simulink model "DLCReferenceApplication"  (R2018a)
settings: Solver=ode23tb  StartTime=0.0  StopTime=20  FixedStep=.001  RelTol=5e-3  EnableMultiTasking=on
StartFcn:
  | %tic
StopFcn:
  | %toc
model workspace (MAT data in the model file):
  A_mu = 10
  B_reff = 8.386
  Cz = 7766.25
  DCT_Param : struct (value not decoded)
  D_reff = 0.25826
  Downshift_Speeds = [9.5625 12.9375 16.3125 19.6875 23.0625 26.4375 29.8125 33.1875 36.5625 39.9375 43.3125 46.6875 ... (28 elements, 4x7)]
  Pedal_Positions = [0.1 0.4 0.5 0.9]
  SUS : struct (value not decoded)
  Upshift_Speeds = [12.9375 16.3125 19.6875 33 26.4375 29.8125 33.1875 52.5 39.9375 43.3125 46.6875 77.25 ... (28 elements, 4x7)]
  VEH : struct (value not decoded)
  V_o = 16.7
  V_xlow = 1
  WH : struct (value not decoded)
  a = 1.4
  alpha_max = 1.5
  alpha_min = -1.5
  b = 1.8
  c_zo = 209651
  epsilon = 0.1
  h = 0.134
  path : struct (value not decoded)
  pio = 220000
  q_Fcx = 0
  q_Fz2 = 15.4
  q_Fzy = 0
  q_reo = 0.9974
  q_sx1 = -0.007764
  q_sx10 = 0.2824
  q_sx11 = 5.349
  q_sx12 = 0
  q_sx13 = 0
  q_sx14 = 0
  q_sx2 = 1.1915
  q_sx3 = 0.013948
  q_sx4 = 4.912
  q_sx5 = 1.02
  q_sx6 = 22.83
  q_sx7 = 0.7104
  q_sx8 = -0.023393
  q_sx9 = 0.6581
  q_sy1 = 0.00702
  q_sy2 = 0
  q_sy3 = 0.001515
  q_sy4 = 8.514e-05
  q_sy5 = 0
  q_sy6 = 0
  q_sy7 = 0.9008
  q_sy8 = -0.4089
  q_v1 = 0.0007742
  q_v2 = 0.04667
  r_Bx1 = 12.531
  r_Bx2 = 9.532
  r_Bx3 = 0
  r_By1 = 10.615
  r_By2 = 7.705
  r_By3 = 3.433e-06
  r_By4 = 0
  r_Cx1 = 1.019
  r_Cy1 = 1.0585
  r_Ex1 = -0.4487
  r_Ex2 = -0.4726
  r_Ey1 = 0.3132
  r_Ey2 = 7.63e-06
  r_Hx1 = 0.0002374
  r_Hy1 = 0.011646
  r_Hy2 = 7.63e-06
  r_Vy1 = 0.05654
  r_Vy2 = 7.63e-06
  r_Vy3 = 0
  r_Vy4 = 99.9
  r_Vy5 = 2
  r_Vy6 = 15.814
  r_o = 0.3135
  vehWidth = 2
  w = 1
symbols that are objects in the model workspace (value not decoded): VEH
libraries: neural x286, simulink x5, sim3dlib x2, autolibutils x1, vehdynlibscenariocommon x1, vehdynlibdriver x1, vehdynlibviscommon x1
(part 8 of 13)

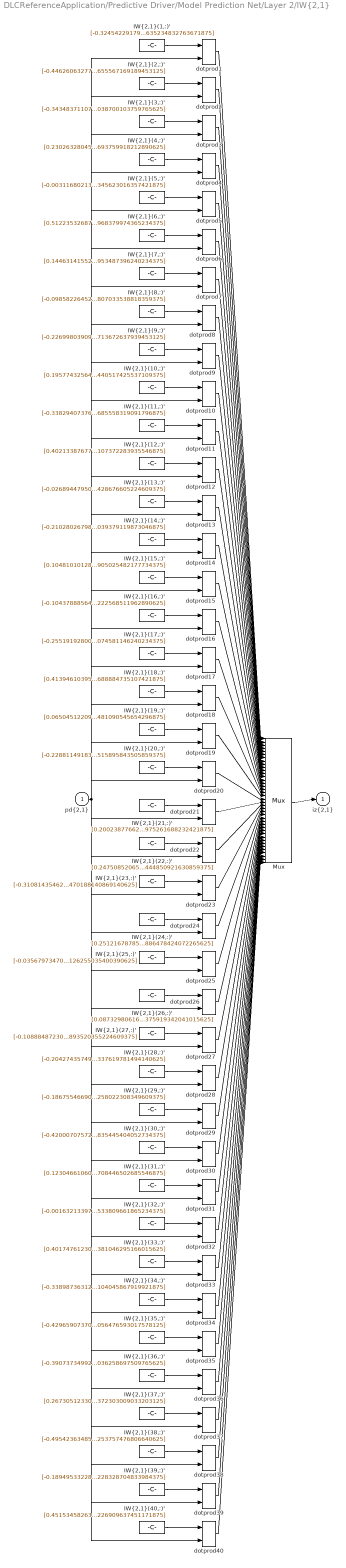
== system DLCReferenceApplication/Predictive Driver/Model Prediction Net/Layer 2/IW{2,1} ==
  "pd{2,1}" : Inport  PortDimensions=9
      mask Display: e = 0.06;c1 = [120 230 180]/255;c2 = ([120 230 180]+0)/(256+128);c3 = ([120 230 180]+128)/(256+128);patch([0 1 1 0],[0 0 1 1],c1);patch([0 1 1 1-e 1-e 0+e],[0 0 1 1-e 0+e 0+e],c2);patch([0 0 1 1-e 0+e 0+e],[0 1 1 1-e 1-e 0+e],c3);plot([0 1 1 0 0],[0 0 1 1 0]);
  "IW{2,1}(1,:)'" : Constant  Value=[-0.324542291796775683732079187393537722527980804443359375;0.0687875470540312006217931184437475167214870452880859375;-0.28041153589947598323561805955250747501850128173828125;0.1679354382406141044103975445977994240820407867431640625;-0.00584034343573799387405731664557606563903391361236572265625;-0.08695050204507125124475663824341609142720699310302734375;-0.37068121178757651446034060427336953580379486083984375;0.63669738948850274073976152067189104855060577392578125;-0.38189062518176353222543184529058635234832763671875]
      mask Display: e = 0.06;c1 = [120 150 230]/255;c2 = ([120 150 230]+0)/383;c3 = ([120 150 230]+128)/383;patch([0 1 1 0],[0 0 1 1],c1);patch([0 1 1 1-e 1-e 0+e],[0 0 1 1-e 0+e 0+e],c2);patch([0 0 1 1-e 0+e 0+e],[0 1 1 1-e 1-e 0+e],c3);plot([0 1 1 0 0],[0 0 1 1 0]);disp('Weights');
  "IW{2,1}(10,:)'" : Constant  Value=[0.1957743256441802082168379683935199864208698272705078125;-0.00790690423303845764391173389640243840403854846954345703125;0.2807004355283073682159056261298246681690216064453125;-0.1709484406753312979443393260226002894341945648193359375;0.1292261121435868409523806121796951629221439361572265625;0.090576606811163140609011179549270309507846832275390625;-0.30742917612599141019558146581402979791164398193359375;0.5389468080432144869718058544094674289226531982421875;-0.355730641305932626661245876675820909440517425537109375]
      mask Display: e = 0.06;c1 = [120 150 230]/255;c2 = ([120 150 230]+0)/383;c3 = ([120 150 230]+128)/383;patch([0 1 1 0],[0 0 1 1],c1);patch([0 1 1 1-e 1-e 0+e],[0 0 1 1-e 0+e 0+e],c2);patch([0 0 1 1-e 0+e 0+e],[0 1 1 1-e 1-e 0+e],c3);plot([0 1 1 0 0],[0 0 1 1 0]);disp('Weights');
  "IW{2,1}(11,:)'" : Constant  Value=[-0.3382940737674229314535523371887393295764923095703125;0.136301301719288614489045130540034733712673187255859375;0.077184732021632618259587843567715026438236236572265625;-0.2946849138566107750847322677145712077617645263671875;0.55020512470717031217048997859819792211055755615234375;0.336723165091655063374531664521782658994197845458984375;-0.496038250235261990450652547224308364093303680419921875;-0.2276057442694929822124549900763668119907379150390625;0.221570869972811113068900112921255640685558319091796875]
      mask Display: e = 0.06;c1 = [120 150 230]/255;c2 = ([120 150 230]+0)/383;c3 = ([120 150 230]+128)/383;patch([0 1 1 0],[0 0 1 1],c1);patch([0 1 1 1-e 1-e 0+e],[0 0 1 1-e 0+e 0+e],c2);patch([0 0 1 1-e 0+e 0+e],[0 1 1 1-e 1-e 0+e],c3);plot([0 1 1 0 0],[0 0 1 1 0]);disp('Weights');
  "IW{2,1}(12,:)'" : Constant  Value=[0.40213387677751477600196494677220471203327178955078125;0.136644910573546829457569629084900952875614166259765625;-0.2578531101404093472950762588880024850368499755859375;0.310418938284677980998793600520002655684947967529296875;-0.4257927265207228639809500236879102885723114013671875;-0.498352245956162509532560989100602455437183380126953125;0.1750266792239182633839078562232316471636295318603515625;-0.00128703269928016048907759572017539539956487715244293212890625;0.49355683974621011866901199027779512107372283935546875]
      mask Display: e = 0.06;c1 = [120 150 230]/255;c2 = ([120 150 230]+0)/383;c3 = ([120 150 230]+128)/383;patch([0 1 1 0],[0 0 1 1],c1);patch([0 1 1 1-e 1-e 0+e],[0 0 1 1-e 0+e 0+e],c2);patch([0 0 1 1-e 0+e 0+e],[0 1 1 1-e 1-e 0+e],c3);plot([0 1 1 0 0],[0 0 1 1 0]);disp('Weights');
  "IW{2,1}(13,:)'" : Constant  Value=[-0.0268944795008402744163067410454459604807198047637939453125;0.160778563268169139011121160365291871130466461181640625;-0.63333375741451813922822111635468900203704833984375;-0.361822351242176265539995938524953089654445648193359375;0.080833836745488218955557613298879005014896392822265625;0.272846015059181545847621919165248982608318328857421875;0.0640400439979145474911348401292343623936176300048828125;-0.4070909764860017876486608656705357134342193603515625;0.2056920660289839053458393891560263000428676605224609375]
      mask Display: e = 0.06;c1 = [120 150 230]/255;c2 = ([120 150 230]+0)/383;c3 = ([120 150 230]+128)/383;patch([0 1 1 0],[0 0 1 1],c1);patch([0 1 1 1-e 1-e 0+e],[0 0 1 1-e 0+e 0+e],c2);patch([0 0 1 1-e 0+e 0+e],[0 1 1 1-e 1-e 0+e],c3);plot([0 1 1 0 0],[0 0 1 1 0]);disp('Weights');
  "IW{2,1}(14,:)'" : Constant  Value=[-0.2102802679827652510002877761507988907396793365478515625;0.3021164324474343576554247192689217627048492431640625;-0.60946876714005371322713244808255694806575775146484375;-0.05831772096079734790663451349246315658092498779296875;0.044852540651126072968057911793948733247816562652587890625;0.51936381618280014205168981789029203355312347412109375;0.39191774273829504959820724252494983375072479248046875;-0.07643630317209677837997361393718165345489978790283203125;0.10716909492530739267390771374266478233039379119873046875]
      mask Display: e = 0.06;c1 = [120 150 230]/255;c2 = ([120 150 230]+0)/383;c3 = ([120 150 230]+128)/383;patch([0 1 1 0],[0 0 1 1],c1);patch([0 1 1 1-e 1-e 0+e],[0 0 1 1-e 0+e 0+e],c2);patch([0 0 1 1-e 0+e 0+e],[0 1 1 1-e 1-e 0+e],c3);plot([0 1 1 0 0],[0 0 1 1 0]);disp('Weights');
  "IW{2,1}(15,:)'" : Constant  Value=[0.10481010128808508630182672050068504177033901214599609375;-0.40408651502036996294719983779941685497760772705078125;0.059323067380531703529644715899848961271345615386962890625;-0.425252943306168251780263744876720011234283447265625;-0.00406918681322654580967412840664110262878239154815673828125;-0.36831496090308790680722950128256343305110931396484375;-0.00676414124778230811674273326161710429005324840545654296875;0.290711580832553939668372322557843290269374847412109375;0.12961919138211808188998475088737905025482177734375]
      mask Display: e = 0.06;c1 = [120 150 230]/255;c2 = ([120 150 230]+0)/383;c3 = ([120 150 230]+128)/383;patch([0 1 1 0],[0 0 1 1],c1);patch([0 1 1 1-e 1-e 0+e],[0 0 1 1-e 0+e 0+e],c2);patch([0 0 1 1-e 0+e 0+e],[0 1 1 1-e 1-e 0+e],c3);plot([0 1 1 0 0],[0 0 1 1 0]);disp('Weights');
  "IW{2,1}(16,:)'" : Constant  Value=[-0.10437888564191878659759282754748710431158542633056640625;0.37692871141585648775418349032406695187091827392578125;-0.11196089219812936643716483331445488147437572479248046875;0.504896824239442043591452602413482964038848876953125;-0.08943749883851202786555489865349954925477504730224609375;-0.59270868880439753212385767255909740924835205078125;0.448211585791503275277847251345519907772541046142578125;0.218911638229702998348358278235537000000476837158203125;0.160338351983476068429723682129406370222568511962890625]
      mask Display: e = 0.06;c1 = [120 150 230]/255;c2 = ([120 150 230]+0)/383;c3 = ([120 150 230]+128)/383;patch([0 1 1 0],[0 0 1 1],c1);patch([0 1 1 1-e 1-e 0+e],[0 0 1 1-e 0+e 0+e],c2);patch([0 0 1 1-e 0+e 0+e],[0 1 1 1-e 1-e 0+e],c3);plot([0 1 1 0 0],[0 0 1 1 0]);disp('Weights');
  "IW{2,1}(17,:)'" : Constant  Value=[-0.25519192800926837616515285844798199832439422607421875;-0.1196708064125363846219585184371680952608585357666015625;-0.06425659036695470505140548311828752048313617706298828125;0.65005912316745007029084035821142606437206268310546875;0.01868941739461237039332530684987432323396205902099609375;0.45198654437769814062875184390577487647533416748046875;-0.11451150435999847554402464311351650394499301910400390625;-0.294471780554158069076464698810013942420482635498046875;0.43042420605367348596104193347855471074581146240234375]
      mask Display: e = 0.06;c1 = [120 150 230]/255;c2 = ([120 150 230]+0)/383;c3 = ([120 150 230]+128)/383;patch([0 1 1 0],[0 0 1 1],c1);patch([0 1 1 1-e 1-e 0+e],[0 0 1 1-e 0+e 0+e],c2);patch([0 0 1 1-e 0+e 0+e],[0 1 1 1-e 1-e 0+e],c3);plot([0 1 1 0 0],[0 0 1 1 0]);disp('Weights');
  "IW{2,1}(18,:)'" : Constant  Value=[0.413946103958608258022167092349263839423656463623046875;-0.398654216100506386677437831167480908334255218505859375;-0.06603405433678495584093326442598481662571430206298828125;-0.335393951206770013495628290911554358899593353271484375;-0.252041180418388577333388411716441623866558074951171875;-0.0492452080997454466615437240761821158230304718017578125;0.1078446964670359553561951315714395605027675628662109375;-0.0245515916688638959064494571293835178948938846588134765625;-0.08793595056549541322254981423611752688884735107421875]
      mask Display: e = 0.06;c1 = [120 150 230]/255;c2 = ([120 150 230]+0)/383;c3 = ([120 150 230]+128)/383;patch([0 1 1 0],[0 0 1 1],c1);patch([0 1 1 1-e 1-e 0+e],[0 0 1 1-e 0+e 0+e],c2);patch([0 0 1 1-e 0+e 0+e],[0 1 1 1-e 1-e 0+e],c3);plot([0 1 1 0 0],[0 0 1 1 0]);disp('Weights');
  "IW{2,1}(19,:)'" : Constant  Value=[0.0650451220991985490371689593303017318248748779296875;-0.473139326014514527418697298344341106712818145751953125;-0.1084104694585747152846266772030503489077091217041015625;0.379416225433231335539829842673498205840587615966796875;0.5098419425723628162216982673271559178829193115234375;0.3359748314586503692424912514979951083660125732421875;0.1408202313841695196838799120087060146033763885498046875;0.044720466722243702728523118139491998590528964996337890625;-0.46815175116202911720364454595255665481090545654296875]
      mask Display: e = 0.06;c1 = [120 150 230]/255;c2 = ([120 150 230]+0)/383;c3 = ([120 150 230]+128)/383;patch([0 1 1 0],[0 0 1 1],c1);patch([0 1 1 1-e 1-e 0+e],[0 0 1 1-e 0+e 0+e],c2);patch([0 0 1 1-e 0+e 0+e],[0 1 1 1-e 1-e 0+e],c3);plot([0 1 1 0 0],[0 0 1 1 0]);disp('Weights');
  "IW{2,1}(2,:)'" : Constant  Value=[-0.4462606327716136522809620146290399134159088134765625;0.1795256506922486838817576426663435995578765869140625;0.07827206229843190754547066489976714365184307098388671875;-0.046401788006822895782388371799243032000958919525146484375;-0.0966140748311935804171213248991989530622959136962890625;-0.405936492152293826318754099702346138656139373779296875;0.454716362534842322151718008171883411705493927001953125;0.286193241696256706063650199212133884429931640625;0.3368045812154509821567671679076738655567169189453125]
      mask Display: e = 0.06;c1 = [120 150 230]/255;c2 = ([120 150 230]+0)/383;c3 = ([120 150 230]+128)/383;patch([0 1 1 0],[0 0 1 1],c1);patch([0 1 1 1-e 1-e 0+e],[0 0 1 1-e 0+e 0+e],c2);patch([0 0 1 1-e 0+e 0+e],[0 1 1 1-e 1-e 0+e],c3);plot([0 1 1 0 0],[0 0 1 1 0]);disp('Weights');
  "IW{2,1}(20,:)'" : Constant  Value=[-0.2288114918340828640719308850748348049819469451904296875;0.2591841189703394388033075301791541278362274169921875;0.0173259779226888899206215910453465767204761505126953125;0.326692029285919394165915718986070714890956878662109375;-0.298978393393575070380308034145855344831943511962890625;0.228846293911817266764074929596972651779651641845703125;0.107487498939770220740541617487906478345394134521484375;-0.100147018257370434834996331119327805936336517333984375;0.2118842852252636743681790676419041119515895843505859375]
      mask Display: e = 0.06;c1 = [120 150 230]/255;c2 = ([120 150 230]+0)/383;c3 = ([120 150 230]+128)/383;patch([0 1 1 0],[0 0 1 1],c1);patch([0 1 1 1-e 1-e 0+e],[0 0 1 1-e 0+e 0+e],c2);patch([0 0 1 1-e 0+e 0+e],[0 1 1 1-e 1-e 0+e],c3);plot([0 1 1 0 0],[0 0 1 1 0]);disp('Weights');
  "IW{2,1}(21,:)'" : Constant  Value=[0.2002387766277574920881221487434231676161289215087890625;0.07527120594866180958160128966483171097934246063232421875;-0.0068731163359172231519522711096215061843395233154296875;0.055941951751786067603688934468664228916168212890625;0.2118083536317571236029522196986363269388675689697265625;0.5015434405608691914579821968800388276576995849609375;0.4018949623650123204043893565540201961994171142578125;-0.08120223725845678031109997618841589428484439849853515625;-0.344831069904761811084625833245809189975261688232421875]
      mask Display: e = 0.06;c1 = [120 150 230]/255;c2 = ([120 150 230]+0)/383;c3 = ([120 150 230]+128)/383;patch([0 1 1 0],[0 0 1 1],c1);patch([0 1 1 1-e 1-e 0+e],[0 0 1 1-e 0+e 0+e],c2);patch([0 0 1 1-e 0+e 0+e],[0 1 1 1-e 1-e 0+e],c3);plot([0 1 1 0 0],[0 0 1 1 0]);disp('Weights');
  "IW{2,1}(22,:)'" : Constant  Value=[0.2475085206523142400403258989172172732651233673095703125;0.23861474844312702270343606869573704898357391357421875;-0.17571858451457689209718182610231451690196990966796875;-0.2493199612004657061969936648893053643405437469482421875;0.07489827097856412152498961631863494403660297393798828125;0.1173975635774616443907092389054014347493648529052734375;-0.543042270824459993860955364652909338474273681640625;-0.326360155936742890592228150126175023615360260009765625;0.004112900763014958570307211260796975693665444850921630859375]
      mask Display: e = 0.06;c1 = [120 150 230]/255;c2 = ([120 150 230]+0)/383;c3 = ([120 150 230]+128)/383;patch([0 1 1 0],[0 0 1 1],c1);patch([0 1 1 1-e 1-e 0+e],[0 0 1 1-e 0+e 0+e],c2);patch([0 0 1 1-e 0+e 0+e],[0 1 1 1-e 1-e 0+e],c3);plot([0 1 1 0 0],[0 0 1 1 0]);disp('Weights');
  "IW{2,1}(23,:)'" : Constant  Value=[-0.310814354629131817109310986779746599495410919189453125;0.72670321668736359566054261449608020484447479248046875;0.255403230644371925794899880202137865126132965087890625;-0.28671289745599659593011665492667816579341888427734375;0.28268366705520919790473044486134313046932220458984375;0.0043791555742623312907912946911892504431307315826416015625;0.158278958994904350721100172449951060116291046142578125;0.01686723224789828112779588309422251768410205841064453125;0.3440386365572809523882824578322470188140869140625]
      mask Display: e = 0.06;c1 = [120 150 230]/255;c2 = ([120 150 230]+0)/383;c3 = ([120 150 230]+128)/383;patch([0 1 1 0],[0 0 1 1],c1);patch([0 1 1 1-e 1-e 0+e],[0 0 1 1-e 0+e 0+e],c2);patch([0 0 1 1-e 0+e 0+e],[0 1 1 1-e 1-e 0+e],c3);plot([0 1 1 0 0],[0 0 1 1 0]);disp('Weights');
  "IW{2,1}(24,:)'" : Constant  Value=[0.251216787859257995041417643733439035713672637939453125;-0.2178828155331899163460462887087487615644931793212890625;0.34863512640181848478704296212526969611644744873046875;-0.4370135838717299492373058455996215343475341796875;0.032467553704689511295811144009348936378955841064453125;0.44547652639035006938428296052734367549419403076171875;-0.474384317933438659498079914556001313030719757080078125;0.288995803879466162111810945134493522346019744873046875;-0.392749260476631667504676670432672835886478424072265625]
      mask Display: e = 0.06;c1 = [120 150 230]/255;c2 = ([120 150 230]+0)/383;c3 = ([120 150 230]+128)/383;patch([0 1 1 0],[0 0 1 1],c1);patch([0 1 1 1-e 1-e 0+e],[0 0 1 1-e 0+e 0+e],c2);patch([0 0 1 1-e 0+e 0+e],[0 1 1 1-e 1-e 0+e],c3);plot([0 1 1 0 0],[0 0 1 1 0]);disp('Weights');
  "IW{2,1}(25,:)'" : Constant  Value=[-0.035679734700623876031411185749675496481359004974365234375;-0.1981953207608193323618905878902296535670757293701171875;-0.06943748085965927019369559047845541499555110931396484375;0.314915993547127348595182638746337033808231353759765625;0.382395395254002179452612608656636439263820648193359375;0.267794186854816318454908241619705222547054290771484375;-0.055846164043513717156752562686961027793586254119873046875;0.2137257342366756518448056567649473436176776885986328125;0.27670835667027626758596170475357212126255035400390625]
      mask Display: e = 0.06;c1 = [120 150 230]/255;c2 = ([120 150 230]+0)/383;c3 = ([120 150 230]+128)/383;patch([0 1 1 0],[0 0 1 1],c1);patch([0 1 1 1-e 1-e 0+e],[0 0 1 1-e 0+e 0+e],c2);patch([0 0 1 1-e 0+e 0+e],[0 1 1 1-e 1-e 0+e],c3);plot([0 1 1 0 0],[0 0 1 1 0]);disp('Weights');
  "IW{2,1}(26,:)'" : Constant  Value=[0.08732980616760983860746847540212911553680896759033203125;-0.13907933838675301529974603909067809581756591796875;-0.2286886511817441125504757337694172747433185577392578125;0.316083898060651236061602276095072738826274871826171875;-0.35283192589203249411866636364720761775970458984375;-0.59883380956851695042786332123796455562114715576171875;-0.549513150841128616974629039759747684001922607421875;-0.058730077914676027950324765924960956908762454986572265625;0.127741615557951659898350271760136820375919342041015625]
      mask Display: e = 0.06;c1 = [120 150 230]/255;c2 = ([120 150 230]+0)/383;c3 = ([120 150 230]+128)/383;patch([0 1 1 0],[0 0 1 1],c1);patch([0 1 1 1-e 1-e 0+e],[0 0 1 1-e 0+e 0+e],c2);patch([0 0 1 1-e 0+e 0+e],[0 1 1 1-e 1-e 0+e],c3);plot([0 1 1 0 0],[0 0 1 1 0]);disp('Weights');
  "IW{2,1}(27,:)'" : Constant  Value=[-0.10888487230919950687901831543058506213128566741943359375;-0.57473736569455591283173134797834791243076324462890625;-0.2335067309102359101036228139491868205368518829345703125;0.2662771068718818856524421789799816906452178955078125;-0.60767973848669043501757869307766668498516082763671875;-0.229561050232402974469181344829848967492580413818359375;-0.70110707356384593946785344087402336299419403076171875;0.275262229425490667633624752852483652532100677490234375;0.312627808227082970571331088649458251893520355224609375]
      mask Display: e = 0.06;c1 = [120 150 230]/255;c2 = ([120 150 230]+0)/383;c3 = ([120 150 230]+128)/383;patch([0 1 1 0],[0 0 1 1],c1);patch([0 1 1 1-e 1-e 0+e],[0 0 1 1-e 0+e 0+e],c2);patch([0 0 1 1-e 0+e 0+e],[0 1 1 1-e 1-e 0+e],c3);plot([0 1 1 0 0],[0 0 1 1 0]);disp('Weights');
  "IW{2,1}(28,:)'" : Constant  Value=[-0.2042743574975654785585987838203436695039272308349609375;0.281950532406683385122647678144858218729496002197265625;0.37992510537679258231236190113122574985027313232421875;-0.268500190748743872148907030350528657436370849609375;-0.65312061664372744740347798142465762794017791748046875;-0.316418870831869980531081409935723058879375457763671875;-0.094265510297374455195296150122885592281818389892578125;-0.3891908495405498324970494650187902152538299560546875;-0.39576383991440666765271316762664355337619781494140625]
      mask Display: e = 0.06;c1 = [120 150 230]/255;c2 = ([120 150 230]+0)/383;c3 = ([120 150 230]+128)/383;patch([0 1 1 0],[0 0 1 1],c1);patch([0 1 1 1-e 1-e 0+e],[0 0 1 1-e 0+e 0+e],c2);patch([0 0 1 1-e 0+e 0+e],[0 1 1 1-e 1-e 0+e],c3);plot([0 1 1 0 0],[0 0 1 1 0]);disp('Weights');
  "IW{2,1}(29,:)'" : Constant  Value=[-0.1867554669027818026183496158409980125725269317626953125;0.43406117590720605381449104243074543774127960205078125;0.09815992793706264374353764878833317197859287261962890625;-0.424804274364632472593683587547275237739086151123046875;0.256399968877172701464672854854143224656581878662109375;0.165621572589895016403005456595565192401409149169921875;0.297412555207232143228424092740169726312160491943359375;0.1337362641868134749412178052807576023042201995849609375;-0.142159918248533079232487352783209644258022308349609375]
      mask Display: e = 0.06;c1 = [120 150 230]/255;c2 = ([120 150 230]+0)/383;c3 = ([120 150 230]+128)/383;patch([0 1 1 0],[0 0 1 1],c1);patch([0 1 1 1-e 1-e 0+e],[0 0 1 1-e 0+e 0+e],c2);patch([0 0 1 1-e 0+e 0+e],[0 1 1 1-e 1-e 0+e],c3);plot([0 1 1 0 0],[0 0 1 1 0]);disp('Weights');
  "IW{2,1}(3,:)'" : Constant  Value=[-0.343483711070276920285238020369433797895908355712890625;0.53066417978020030687957842019386589527130126953125;0.31171502011341678528566490058437921106815338134765625;-0.444047795862383465337330790134728886187076568603515625;0.236383550289809674094243518993607722222805023193359375;-0.334990509854110107834657128478283993899822235107421875;0.256484526856124606108977559415507130324840545654296875;0.0082278378919732504670481176844987203367054462432861328125;0.325626509224444637968787219506339170038700103759765625]
      mask Display: e = 0.06;c1 = [120 150 230]/255;c2 = ([120 150 230]+0)/383;c3 = ([120 150 230]+128)/383;patch([0 1 1 0],[0 0 1 1],c1);patch([0 1 1 1-e 1-e 0+e],[0 0 1 1-e 0+e 0+e],c2);patch([0 0 1 1-e 0+e 0+e],[0 1 1 1-e 1-e 0+e],c3);plot([0 1 1 0 0],[0 0 1 1 0]);disp('Weights');
  "IW{2,1}(30,:)'" : Constant  Value=[-0.420007075724736667066139261805801652371883392333984375;-0.325973267627817531177925047813914716243743896484375;-0.45662813284732284291322912395116873085498809814453125;-0.2121125175206574342556820056415745057165622711181640625;0.388440219381910589735440453296178020536899566650390625;-0.4829169636928585251922640964039601385593414306640625;0.2238460597286293929375489142330479808151721954345703125;-0.0248133086022019784533387820602001738734543323516845703125;0.0229742725381577549137457339156753732822835445404052734375]
      mask Display: e = 0.06;c1 = [120 150 230]/255;c2 = ([120 150 230]+0)/383;c3 = ([120 150 230]+128)/383;patch([0 1 1 0],[0 0 1 1],c1);patch([0 1 1 1-e 1-e 0+e],[0 0 1 1-e 0+e 0+e],c2);patch([0 0 1 1-e 0+e 0+e],[0 1 1 1-e 1-e 0+e],c3);plot([0 1 1 0 0],[0 0 1 1 0]);disp('Weights');
  "IW{2,1}(31,:)'" : Constant  Value=[0.12304661060634934643953641852931468747556209564208984375;0.0935386299662377129759960325827705673873424530029296875;-0.313172631359989572796820311850751750171184539794921875;-0.37907455437369852457862862138426862657070159912109375;-0.32895518023903924653694730295683257281780242919921875;0.150482777563526404218663401479716412723064422607421875;-0.25216581763143597338938661778229288756847381591796875;-0.352642844402300259520899317067232914268970489501953125;0.14167340657996163599818828515708446502685546875]
      mask Display: e = 0.06;c1 = [120 150 230]/255;c2 = ([120 150 230]+0)/383;c3 = ([120 150 230]+128)/383;patch([0 1 1 0],[0 0 1 1],c1);patch([0 1 1 1-e 1-e 0+e],[0 0 1 1-e 0+e 0+e],c2);patch([0 0 1 1-e 0+e 0+e],[0 1 1 1-e 1-e 0+e],c3);plot([0 1 1 0 0],[0 0 1 1 0]);disp('Weights');
  "IW{2,1}(32,:)'" : Constant  Value=[-0.00163213397447740222144518806857149684219621121883392333984375;-0.206420648244373172719434705868479795753955841064453125;0.0098161331607758035844302213490664144046604633331298828125;0.1949452791234642656803544014110229909420013427734375;0.35469101103357203452759449646691791713237762451171875;0.047329873783093660832843596608654479496181011199951171875;0.2484372937853538687580368105045636184513568878173828125;0.11516084718418313770360583703222800977528095245361328125;0.20834742157546182195204664822085760533809661865234375]
      mask Display: e = 0.06;c1 = [120 150 230]/255;c2 = ([120 150 230]+0)/383;c3 = ([120 150 230]+128)/383;patch([0 1 1 0],[0 0 1 1],c1);patch([0 1 1 1-e 1-e 0+e],[0 0 1 1-e 0+e 0+e],c2);patch([0 0 1 1-e 0+e 0+e],[0 1 1 1-e 1-e 0+e],c3);plot([0 1 1 0 0],[0 0 1 1 0]);disp('Weights');
  "IW{2,1}(33,:)'" : Constant  Value=[0.401747612301919299060415369240217842161655426025390625;-0.45277690869865150347095550387166440486907958984375;0.395869712515088512105876361601985991001129150390625;0.4756958338025290000672384849167428910732269287109375;0.05436458869313125219502325080611626617610454559326171875;-0.12254264973859607668060789364972151815891265869140625;0.5336371688040433269861750886775553226470947265625;0.42723568675965972740726783740683458745479583740234375;0.28361631892452321412889659768552519381046295166015625]
      mask Display: e = 0.06;c1 = [120 150 230]/255;c2 = ([120 150 230]+0)/383;c3 = ([120 150 230]+128)/383;patch([0 1 1 0],[0 0 1 1],c1);patch([0 1 1 1-e 1-e 0+e],[0 0 1 1-e 0+e 0+e],c2);patch([0 0 1 1-e 0+e 0+e],[0 1 1 1-e 1-e 0+e],c3);plot([0 1 1 0 0],[0 0 1 1 0]);disp('Weights');
  "IW{2,1}(34,:)'" : Constant  Value=[-0.33898736312202981668662005176884122192859649658203125;0.01404114771738000817802305419945696485228836536407470703125;0.1980737895577827367699086380525841377675533294677734375;0.06345794786319562674758998355173389427363872528076171875;0.490762924647671849864849491495988331735134124755859375;-0.51565340020439565105192514238297007977962493896484375;-0.284663969744654077320689111729734577238559722900390625;-0.404971717505282213789286061000893823802471160888671875;-0.1739486054948659876639993626668001525104045867919921875]
      mask Display: e = 0.06;c1 = [120 150 230]/255;c2 = ([120 150 230]+0)/383;c3 = ([120 150 230]+128)/383;patch([0 1 1 0],[0 0 1 1],c1);patch([0 1 1 1-e 1-e 0+e],[0 0 1 1-e 0+e 0+e],c2);patch([0 0 1 1-e 0+e 0+e],[0 1 1 1-e 1-e 0+e],c3);plot([0 1 1 0 0],[0 0 1 1 0]);disp('Weights');
  "IW{2,1}(35,:)'" : Constant  Value=[-0.429659073706359306843438616851926781237125396728515625;-0.1784271749077228907953696079857763834297657012939453125;0.440909793280942874371675088696065358817577362060546875;-0.442994791296781154077422115733497776091098785400390625;-0.019944572767950190239627517030385206453502178192138671875;-0.03606031173514055720996651643872610293328762054443359375;0.540340210876711690701768020517192780971527099609375;0.1381670843642019141928045655731693841516971588134765625;0.496062396810801609081664764744346030056476593017578125]
      mask Display: e = 0.06;c1 = [120 150 230]/255;c2 = ([120 150 230]+0)/383;c3 = ([120 150 230]+128)/383;patch([0 1 1 0],[0 0 1 1],c1);patch([0 1 1 1-e 1-e 0+e],[0 0 1 1-e 0+e 0+e],c2);patch([0 0 1 1-e 0+e 0+e],[0 1 1 1-e 1-e 0+e],c3);plot([0 1 1 0 0],[0 0 1 1 0]);disp('Weights');
  "IW{2,1}(36,:)'" : Constant  Value=[-0.39073734992504605134655548681621439754962921142578125;-0.303381329616073502908335512984194792807102203369140625;0.004042519886493571752705822319740036618895828723907470703125;0.266183250969649398687266739216283895075321197509765625;0.18023920737041565498515183207928203046321868896484375;0.296769017276363122892490764570538885891437530517578125;0.39109693442211368452632314074435271322727203369140625;0.03950743425914644835206246398229268379509449005126953125;0.09219891966973338404134352686014608480036258697509765625]
      mask Display: e = 0.06;c1 = [120 150 230]/255;c2 = ([120 150 230]+0)/383;c3 = ([120 150 230]+128)/383;patch([0 1 1 0],[0 0 1 1],c1);patch([0 1 1 1-e 1-e 0+e],[0 0 1 1-e 0+e 0+e],c2);patch([0 0 1 1-e 0+e 0+e],[0 1 1 1-e 1-e 0+e],c3);plot([0 1 1 0 0],[0 0 1 1 0]);disp('Weights');
  "IW{2,1}(37,:)'" : Constant  Value=[0.2673051233086429778751380581525154411792755126953125;-0.50684067738421945126248147062142379581928253173828125;0.177671067497580548177893433603458106517791748046875;0.057268097089858659154426590021103038452565670013427734375;-0.180493895501149304028132291932706721127033233642578125;-0.362951249171143019989216327303438447415828704833984375;0.418656006562284799255024836384109221398830413818359375;-0.204769049504260058913729380947188474237918853759765625;-0.41369900997950292964588925315183587372303009033203125]
      mask Display: e = 0.06;c1 = [120 150 230]/255;c2 = ([120 150 230]+0)/383;c3 = ([120 150 230]+128)/383;patch([0 1 1 0],[0 0 1 1],c1);patch([0 1 1 1-e 1-e 0+e],[0 0 1 1-e 0+e 0+e],c2);patch([0 0 1 1-e 0+e 0+e],[0 1 1 1-e 1-e 0+e],c3);plot([0 1 1 0 0],[0 0 1 1 0]);disp('Weights');
  "IW{2,1}(38,:)'" : Constant  Value=[-0.495423634851604732798335817278712056577205657958984375;0.2043341907914952015890008851783932186663150787353515625;-0.467174720166877610605382642461336217820644378662109375;0.1438508111957102764133509253952070139348506927490234375;-0.1568346784385365733083261829960974864661693572998046875;0.07396871999577396550318297840931336395442485809326171875;0.27031216667364443839716159345698542892932891845703125;-0.2451526543714712957910961677043815143406391143798828125;-0.014373142866274980777863135017469176091253757476806640625]
      mask Display: e = 0.06;c1 = [120 150 230]/255;c2 = ([120 150 230]+0)/383;c3 = ([120 150 230]+128)/383;patch([0 1 1 0],[0 0 1 1],c1);patch([0 1 1 1-e 1-e 0+e],[0 0 1 1-e 0+e 0+e],c2);patch([0 0 1 1-e 0+e 0+e],[0 1 1 1-e 1-e 0+e],c3);plot([0 1 1 0 0],[0 0 1 1 0]);disp('Weights');
  "IW{2,1}(39,:)'" : Constant  Value=[-0.189495332287297368889511517409118823707103729248046875;-0.047299852000780163996385141444989130832254886627197265625;0.1431300344219219311536761551906238310039043426513671875;0.312383402635927176493879642293904908001422882080078125;-0.1039185124131432325089718915478442795574665069580078125;0.277625194286385712505449419040814973413944244384765625;0.2369613096830224530098263358013355173170566558837890625;0.384774011692236239667863628710620105266571044921875;-0.043397234031065178017083638906115083955228328704833984375]
      mask Display: e = 0.06;c1 = [120 150 230]/255;c2 = ([120 150 230]+0)/383;c3 = ([120 150 230]+128)/383;patch([0 1 1 0],[0 0 1 1],c1);patch([0 1 1 1-e 1-e 0+e],[0 0 1 1-e 0+e 0+e],c2);patch([0 0 1 1-e 0+e 0+e],[0 1 1 1-e 1-e 0+e],c3);plot([0 1 1 0 0],[0 0 1 1 0]);disp('Weights');
  "IW{2,1}(4,:)'" : Constant  Value=[0.2302632804560506285529442038750858046114444732666015625;0.056426691973135344182477268759612343274056911468505859375;0.26981815992925073377506350880139507353305816650390625;0.0627338958160852666612328221162897534668445587158203125;-0.0541004381655196819878028691164217889308929443359375;0.07336591425450332548674481358830234967172145843505859375;-0.29929722601775610169028141172020696103572845458984375;0.058258801046390924771589681085970369167625904083251953125;0.624129896202314515818443396710790693759918212890625]
      mask Display: e = 0.06;c1 = [120 150 230]/255;c2 = ([120 150 230]+0)/383;c3 = ([120 150 230]+128)/383;patch([0 1 1 0],[0 0 1 1],c1);patch([0 1 1 1-e 1-e 0+e],[0 0 1 1-e 0+e 0+e],c2);patch([0 0 1 1-e 0+e 0+e],[0 1 1 1-e 1-e 0+e],c3);plot([0 1 1 0 0],[0 0 1 1 0]);disp('Weights');
  "IW{2,1}(40,:)'" : Constant  Value=[0.45153458263285661811181626035249792039394378662109375;0.273234019873488886975820832958561368286609649658203125;0.058358325260174377657751421111242962069809436798095703125;-0.24921725789550486229728676335071213543415069580078125;-0.056418061624276892584983755796201876364648342132568359375;-0.288169974372767312420506868875236250460147857666015625;0.370481762537899383946893294705660082399845123291015625;0.170917408646739599209496418552589602768421173095703125;0.084260395075418770272079882488469593226909637451171875]
      mask Display: e = 0.06;c1 = [120 150 230]/255;c2 = ([120 150 230]+0)/383;c3 = ([120 150 230]+128)/383;patch([0 1 1 0],[0 0 1 1],c1);patch([0 1 1 1-e 1-e 0+e],[0 0 1 1-e 0+e 0+e],c2);patch([0 0 1 1-e 0+e 0+e],[0 1 1 1-e 1-e 0+e],c3);plot([0 1 1 0 0],[0 0 1 1 0]);disp('Weights');
  "IW{2,1}(5,:)'" : Constant  Value=[-0.0031168021329519741968727686298734624870121479034423828125;0.328002271778910670096962576280930079519748687744140625;0.38247228553464041045373278393526561558246612548828125;0.178224480049883116095088553265668451786041259765625;0.1542419981506792936443162034265697002410888671875;-0.283971671856202256822854224083130247890949249267578125;0.11580051943021670013411750232990016229450702667236328125;0.189974925141610129220026692564715631306171417236328125;0.3846379017252352650046987037057988345623016357421875]
      mask Display: e = 0.06;c1 = [120 150 230]/255;c2 = ([120 150 230]+0)/383;c3 = ([120 150 230]+128)/383;patch([0 1 1 0],[0 0 1 1],c1);patch([0 1 1 1-e 1-e 0+e],[0 0 1 1-e 0+e 0+e],c2);patch([0 0 1 1-e 0+e 0+e],[0 1 1 1-e 1-e 0+e],c3);plot([0 1 1 0 0],[0 0 1 1 0]);disp('Weights');
  "IW{2,1}(6,:)'" : Constant  Value=[0.51223532687983708289181095096864737570285797119140625;-0.332082772295919870231273307581432163715362548828125;0.1275842036868156947893027108875685371458530426025390625;-0.379699503766440737972942542910459451377391815185546875;0.2690175410241992803861421634792350232601165771484375;-0.0154989389606303602786585571493560564704239368438720703125;0.158626842633787401570799602268380112946033477783203125;0.50383707239248221032568153532338328659534454345703125;-0.0224399158307635425424475528188850148580968379974365234375]
      mask Display: e = 0.06;c1 = [120 150 230]/255;c2 = ([120 150 230]+0)/383;c3 = ([120 150 230]+128)/383;patch([0 1 1 0],[0 0 1 1],c1);patch([0 1 1 1-e 1-e 0+e],[0 0 1 1-e 0+e 0+e],c2);patch([0 0 1 1-e 0+e 0+e],[0 1 1 1-e 1-e 0+e],c3);plot([0 1 1 0 0],[0 0 1 1 0]);disp('Weights');
  "IW{2,1}(7,:)'" : Constant  Value=[0.1446314155234941500882683840245590545237064361572265625;0.2732545567729920410471322611556388437747955322265625;-0.247854486607387569652161118938238359987735748291015625;0.1630082571171082295169441067628213204443454742431640625;0.436201058352217729829902737037627957761287689208984375;0.05221461830264105541399288767934194765985012054443359375;-0.5396479904293298712758542023948393762111663818359375;-0.135598603508195025835192382146487943828105926513671875;0.51423077506378100931527797001763246953487396240234375]
      mask Display: e = 0.06;c1 = [120 150 230]/255;c2 = ([120 150 230]+0)/383;c3 = ([120 150 230]+128)/383;patch([0 1 1 0],[0 0 1 1],c1);patch([0 1 1 1-e 1-e 0+e],[0 0 1 1-e 0+e 0+e],c2);patch([0 0 1 1-e 0+e 0+e],[0 1 1 1-e 1-e 0+e],c3);plot([0 1 1 0 0],[0 0 1 1 0]);disp('Weights');
  "IW{2,1}(8,:)'" : Constant  Value=[-0.09858226452668465700224231795800733380019664764404296875;0.356305635376591267604595714146853424608707427978515625;0.25550733449753215698052599691436626017093658447265625;0.034878811141299918829883353055265615694224834442138671875;0.304494445379197398171555732915294356644153594970703125;0.09943805056925204832740661231582635082304477691650390625;0.5768483712525982465280094402260147035121917724609375;0.6931058447080447049160056849359534680843353271484375;0.161953318977365368080967300556949339807033538818359375]
      mask Display: e = 0.06;c1 = [120 150 230]/255;c2 = ([120 150 230]+0)/383;c3 = ([120 150 230]+128)/383;patch([0 1 1 0],[0 0 1 1],c1);patch([0 1 1 1-e 1-e 0+e],[0 0 1 1-e 0+e 0+e],c2);patch([0 0 1 1-e 0+e 0+e],[0 1 1 1-e 1-e 0+e],c3);plot([0 1 1 0 0],[0 0 1 1 0]);disp('Weights');
  "IW{2,1}(9,:)'" : Constant  Value=[-0.2269980390922531066077993955332203768193721771240234375;-0.1662544585091897120232573570319800637662410736083984375;-0.1624782913689543917268309769497136585414409637451171875;-0.56136775947428418920281956161488778889179229736328125;0.494008889276872864559919662497122772037982940673828125;-0.302455999625720561851949241827242076396942138671875;-0.1236619127196121048495314198589767329394817352294921875;0.02226648258436135507931652455226867459714412689208984375;-0.51760600642985554742381282267160713672637939453125]
      mask Display: e = 0.06;c1 = [120 150 230]/255;c2 = ([120 150 230]+0)/383;c3 = ([120 150 230]+128)/383;patch([0 1 1 0],[0 0 1 1],c1);patch([0 1 1 1-e 1-e 0+e],[0 0 1 1-e 0+e 0+e],c2);patch([0 0 1 1-e 0+e 0+e],[0 1 1 1-e 1-e 0+e],c3);plot([0 1 1 0 0],[0 0 1 1 0]);disp('Weights');
  Mux : Mux  Inputs=40
      mask Display: e = 0.06;c1 = [120 150 230]/255;c2 = ([120 150 230]+0)/383;c3 = ([120 150 230]+128)/383;patch([0 1 1 0],[0 0 1 1],c1);patch([0 1 1 1-e 1-e 0+e],[0 0 1 1-e 0+e 0+e],c2);patch([0 0 1 1-e 0+e 0+e],[0 1 1 1-e 1-e 0+e],c3);plot([0 1 1 0 0],[0 0 1 1 0]);disp('Mux');
  dotprod{1..40} (40 alike) : neural/Weight Functions/dotprod
  "iz{2,1}" : Outport
      mask Display: e = 0.06;c1 = [120 230 180]/255;c2 = ([120 230 180]+0)/(256+128);c3 = ([120 230 180]+128)/(256+128);patch([0 1 1 0],[0 0 1 1],c1);patch([0 1 1 1-e 1-e 0+e],[0 0 1 1-e 0+e 0+e],c2);patch([0 0 1 1-e 0+e 0+e],[0 1 1 1-e 1-e 0+e],c3);plot([0 1 1 0 0],[0 0 1 1 0]);
  wires:
  "IW{2,1}(1,:)'"/1 -> dotprod1/1
  "pd{2,1}"/1 -> dotprod1/2, dotprod2/2, dotprod3/2, dotprod4/2, dotprod5/2, dotprod6/2, dotprod7/2, dotprod8/2, dotprod9/2, dotprod10/2, dotprod11/2, dotprod12/2, dotprod13/2, dotprod14/2, dotprod15/2, dotprod16/2, dotprod17/2, dotprod18/2, dotprod19/2, dotprod20/2, dotprod21/2, dotprod22/2, dotprod23/2, dotprod24/2, dotprod25/2, dotprod26/2, dotprod27/2, dotprod28/2, dotprod29/2, dotprod30/2, dotprod31/2, dotprod32/2, dotprod33/2, dotprod34/2, dotprod35/2, dotprod36/2, dotprod37/2, dotprod38/2, dotprod39/2, dotprod40/2
  dotprod1/1 -> Mux/1
  "IW{2,1}(2,:)'"/1 -> dotprod2/1
  dotprod2/1 -> Mux/2
  "IW{2,1}(3,:)'"/1 -> dotprod3/1
  dotprod3/1 -> Mux/3
  "IW{2,1}(4,:)'"/1 -> dotprod4/1
  dotprod4/1 -> Mux/4
  "IW{2,1}(5,:)'"/1 -> dotprod5/1
  dotprod5/1 -> Mux/5
  "IW{2,1}(6,:)'"/1 -> dotprod6/1
  dotprod6/1 -> Mux/6
  "IW{2,1}(7,:)'"/1 -> dotprod7/1
  dotprod7/1 -> Mux/7
  "IW{2,1}(8,:)'"/1 -> dotprod8/1
  dotprod8/1 -> Mux/8
  "IW{2,1}(9,:)'"/1 -> dotprod9/1
  dotprod9/1 -> Mux/9
  "IW{2,1}(10,:)'"/1 -> dotprod10/1
  dotprod10/1 -> Mux/10
  "IW{2,1}(11,:)'"/1 -> dotprod11/1
  dotprod11/1 -> Mux/11
  "IW{2,1}(12,:)'"/1 -> dotprod12/1
  dotprod12/1 -> Mux/12
  "IW{2,1}(13,:)'"/1 -> dotprod13/1
  dotprod13/1 -> Mux/13
  "IW{2,1}(14,:)'"/1 -> dotprod14/1
  dotprod14/1 -> Mux/14
  "IW{2,1}(15,:)'"/1 -> dotprod15/1
  dotprod15/1 -> Mux/15
  "IW{2,1}(16,:)'"/1 -> dotprod16/1
  dotprod16/1 -> Mux/16
  "IW{2,1}(17,:)'"/1 -> dotprod17/1
  dotprod17/1 -> Mux/17
  "IW{2,1}(18,:)'"/1 -> dotprod18/1
  dotprod18/1 -> Mux/18
  "IW{2,1}(19,:)'"/1 -> dotprod19/1
  dotprod19/1 -> Mux/19
  "IW{2,1}(20,:)'"/1 -> dotprod20/1
  dotprod20/1 -> Mux/20
  "IW{2,1}(21,:)'"/1 -> dotprod21/1
  dotprod21/1 -> Mux/21
  "IW{2,1}(22,:)'"/1 -> dotprod22/1
  dotprod22/1 -> Mux/22
  "IW{2,1}(23,:)'"/1 -> dotprod23/1
  dotprod23/1 -> Mux/23
  "IW{2,1}(24,:)'"/1 -> dotprod24/1
  dotprod24/1 -> Mux/24
  "IW{2,1}(25,:)'"/1 -> dotprod25/1
  dotprod25/1 -> Mux/25
  "IW{2,1}(26,:)'"/1 -> dotprod26/1
  dotprod26/1 -> Mux/26
  "IW{2,1}(27,:)'"/1 -> dotprod27/1
  dotprod27/1 -> Mux/27
  "IW{2,1}(28,:)'"/1 -> dotprod28/1
  dotprod28/1 -> Mux/28
  "IW{2,1}(29,:)'"/1 -> dotprod29/1
  dotprod29/1 -> Mux/29
  "IW{2,1}(30,:)'"/1 -> dotprod30/1
  dotprod30/1 -> Mux/30
  "IW{2,1}(31,:)'"/1 -> dotprod31/1
  dotprod31/1 -> Mux/31
  "IW{2,1}(32,:)'"/1 -> dotprod32/1
  dotprod32/1 -> Mux/32
  "IW{2,1}(33,:)'"/1 -> dotprod33/1
  dotprod33/1 -> Mux/33
  "IW{2,1}(34,:)'"/1 -> dotprod34/1
  dotprod34/1 -> Mux/34
  "IW{2,1}(35,:)'"/1 -> dotprod35/1
  dotprod35/1 -> Mux/35
  "IW{2,1}(36,:)'"/1 -> dotprod36/1
  dotprod36/1 -> Mux/36
  "IW{2,1}(37,:)'"/1 -> dotprod37/1
  dotprod37/1 -> Mux/37
  "IW{2,1}(38,:)'"/1 -> dotprod38/1
  dotprod38/1 -> Mux/38
  "IW{2,1}(39,:)'"/1 -> dotprod39/1
  dotprod39/1 -> Mux/39
  "IW{2,1}(40,:)'"/1 -> dotprod40/1
  dotprod40/1 -> Mux/40
  Mux/1 -> "iz{2,1}"/1
